simulink model "echo_delay"  (R2024b)
settings: Solver=VariableStepAuto  StartTime=0.0  StopTime=100  RelTol=1e-3
libraries: audiosources x1, dspsnks4 x1
settings Model: Creator=woutlyen  LastModifiedBy=woutlyen

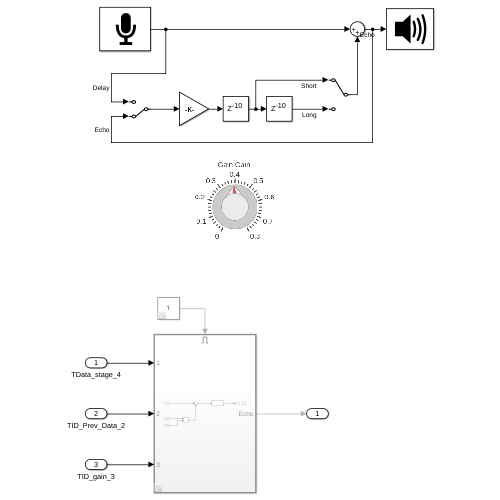
[thumbnail: Simulink's stored preview of the top-level diagram]
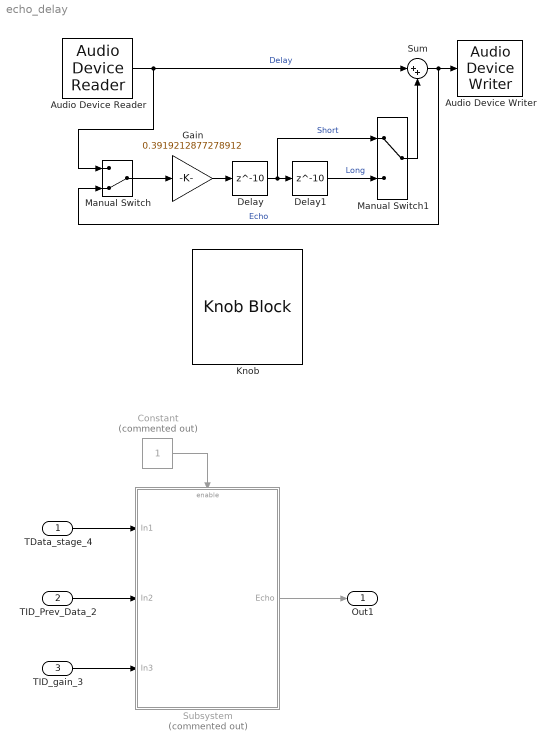
== system echo_delay ==
  TData_stage_4 : Inport  OutDataTypeStr=fixdt(1,24,23)
  TID_Prev_Data_2 : Inport  Port=2  OutDataTypeStr=fixdt(1,24,23)
  TID_gain_3 : Inport  Port=3
  Audio Device Reader : audiosources/Audio Device Reader  Driver=ALSA  Device=Default  SampleRate=44100  NumChannels=1  SamplesPerFrame=1024  BitDepth=16-bit integer  NumBuffers=10  DefaultInputChannelMapping=on  InputChannelMapping=1:2  OutputNumOverrunSamples=off  OutputDataType=double  DriverIdx=8  DeviceWarnFlag=''
  Audio Device Writer : dspsnks4/Audio Device Writer  Driver=ALSA  Device=Default  InheritSampleRate=on  SampleRate=44100  BitDepth=16-bit integer  BufferSize=4096  NumBuffers=10  DefaultOutputChannelMapping=on  OutputChannelMapping=1:2  OutputNumUnderrunSamples=off  DriverIdx=8  DeviceWarnFlag=''
  Constant : Constant  Commented=on  OutDataTypeStr=boolean
  Delay : Delay  DelayLength=10  InitialCondition=0
  Delay1 : Delay  DelayLength=10  InitialCondition=0
  Gain : Gain  Gain=0.3919212877278912
  Knob : KnobBlock  ScaleMax=0.8
  Manual Switch : ManualSwitch  CurrentSetting=0
  Manual Switch1 : ManualSwitch
  Subsystem : Subsystem  Commented=on
  Sum : Sum  Inputs=|++
  Out1 : Outport  VectorParamsAs1DForOutWhenUnconnected=off
  wires:
  Audio Device Reader/1 -> Manual Switch/1, Sum/1  "Delay"
  Gain/1 -> Delay/1
  Delay/1 -> Manual Switch1/1, Delay1/1  "Short"
  Sum/1 -> Manual Switch/2, Audio Device Writer/1  "Echo"
  Manual Switch/1 -> Gain/1
  Delay1/1 -> Manual Switch1/2  "Long"
  Manual Switch1/1 -> Sum/2
  TData_stage_4/1 -> Subsystem/1(In1)
  TID_Prev_Data_2/1 -> Subsystem/2(In2)
  TID_gain_3/1 -> Subsystem/3(In3)
  Subsystem/1(Echo) -> Out1/1
  Constant/1 -> Subsystem/Enable

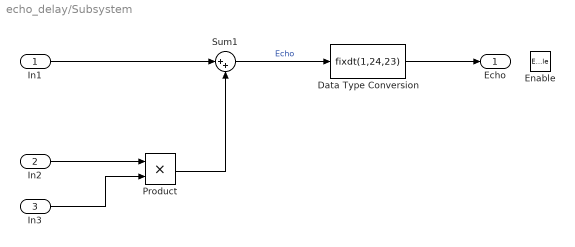
== system echo_delay/Subsystem ==
  In1 : Inport
  In2 : Inport  Port=2
  In3 : Inport  Port=3
  Enable : EnablePort
  Data Type Conversion : DataTypeConversion  OutDataTypeStr=fixdt(1,24,23)  SaturateOnIntegerOverflow=off  RndMeth=Floor
  Product : Product
  Sum1 : Sum  Inputs=|++
  Echo : Outport
  wires:
  Product/1 -> Sum1/2
  In3/1 -> Product/2
  In1/1 -> Sum1/1
  In2/1 -> Product/1
  Sum1/1 -> Data Type Conversion/1  "Echo"
  Data Type Conversion/1 -> Echo/1
